simulink model "verify_Collector_Unglazed_CONF_mdl"  (R2016b)
settings: Solver=ode45  StartTime=0  StopTime=24*3600  MaxStep=600  RelTol=1e-3  EnableMultiTasking=on
InitFcn:
  | load('DE_TRY2010_13_averageYear')
undefined symbols (not defined in the file or in its folder): path_carnot
libraries: carnot x4
settings Model: Creator=drhf  LastModifiedBy=drhf
settings DataIOCC: SaveFormat=Array  SignalLoggingSaveFormat=ModelDataLogs
settings OptimizationCC: ExpressionDepthLimit=2147483647  LifeSpan=inf
settings DebuggingCC: UnderspecifiedInitializationDetection=Classic  MergeDetectMultiDrivingBlocksExec=none  SolverPrmCheckMsg=warning  FcnCallInpInsideContextMsg=warning  StateNameClashWarn=warning  SFUnexpectedBacktrackingDiag=warning  SFNoUnconditionalDefaultTransitionDiag=warning  SFExecutionAtInitializationDiag=none
settings HardwareCC: ProdBitPerPointer=32  ProdBitPerSizeT=32  ProdBitPerPtrDiffT=32  ProdLargestAtomicFloat=None  ProdIntDivRoundTo=Undefined  ProdEndianess=Unspecified  ProdWordSize=32  ProdHWDeviceType=32-bit Generic
settings ModelReferenceCC: PropagateSignalLabelsOutOfModel=off
settings GRTTargetCC: TargetLangStandard=C89/C90 (ANSI)  GeneratePreprocessorConditionals=Disable all  CombineOutputUpdateFcns=off  GRTInterface=on
settings ConfigComp: CovMetricSettings=dw  CovHtmlReporting=on  CovSaveCumulativeToWorkspaceVar=on  CovSaveSingleToWorkspaceVar=on  CovExternalEMLEnable=off

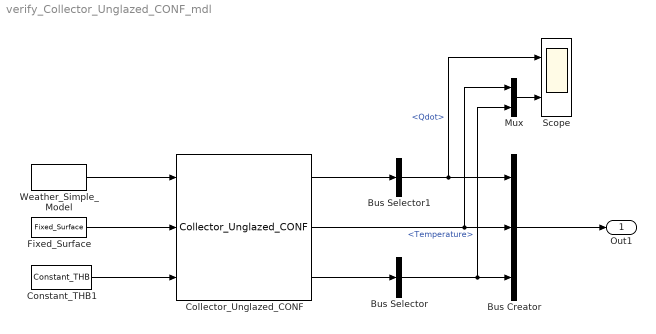
== system verify_Collector_Unglazed_CONF_mdl ==
  Bus Creator : BusCreator  Inputs=3
  Bus Selector : BusSelector  OutputSignals=Temperature
  Bus Selector1 : BusSelector  OutputSignals=Qdot
  Collector_Unglazed_CONF : carnot/Source/Solar_Thermal/Collector_Unglazed_CONF  tini=20  Ncollector=1  PathName=fullfile(path_carnot('libsl'),'Source','Solar_Thermal','Collector_Unglazed_CONF','parameter_set')  FileName='DefaultCollectorUnglazed.mat'  userPath=off  userParam=off  acol=2.5  len=2.3  nodes=5  fta=0.75  eps=0.9  u0l=4  u0c=10  u0g=4  u1l=3  u1c=3  u1g=1.5  u1e=0.01  hi=100  capa=7000  capf=2000  SensorTimeConstant=10  dplin=10  dpqua=10
  Constant_THB1 : carnot/Source/Simple/Constant_THB  t=40  mdot=100/3600  p=1e5  mID=No Pressure Drop  fluid=Water  mix=0  mix2=0  mix3=0  dia=0.02  hgt=0
  Fixed_Surface : carnot/Weather/Fixed_Surface  colangle=30  colazi=0  colrot=0
  Mux : Mux  Inputs=2
  Scope : Scope  NumInputPorts=2
  Weather_Simple_Model : carnot/Weather/Weather_Simple_Model  lat=60  Ibn=900  Idg=100  tamb=5  deltaTsky=-6  rh=50  precip="10e-3/24/3600           % 10 mm in 24 h"  cloud=0.125  p=1013e2  vw=1  wdir=270
  Out1 : Outport
  wires:
  Bus Creator/1 -> Out1/1
  Weather_Simple_Model/1 -> Collector_Unglazed_CONF/1
  Constant_THB1/1 -> Collector_Unglazed_CONF/3
  Fixed_Surface/1 -> Collector_Unglazed_CONF/2
  Collector_Unglazed_CONF/1 -> Bus Selector1/1
  Bus Selector/1 -> Mux/2, Bus Creator/3  "<Temperature>"
  Bus Selector1/1 -> Bus Creator/1, Scope/1  "<Qdot>"
  Collector_Unglazed_CONF/3 -> Bus Selector/1
  Collector_Unglazed_CONF/2 -> Mux/1, Bus Creator/2
  Mux/1 -> Scope/2
